simulink model "tutorial25_simscape"  (R2025a)
settings: Solver=VariableStepAuto  StartTime=0.0  StopTime=10  RelTol=1e-3
settings Model: Creator=xing2  LastModifiedBy=xing2

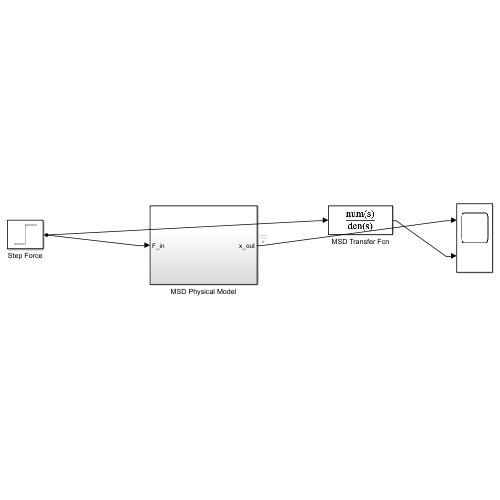
[thumbnail: Simulink's stored preview of the top-level diagram]
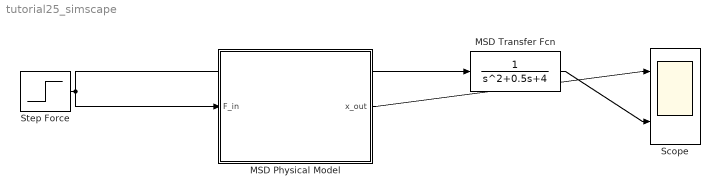
== system tutorial25_simscape ==
  MSD Physical Model : Subsystem
  MSD Transfer Fcn : TransferFcn  Denominator=[1 0.5 4]
  Scope : Scope  NumInputPorts=2
  Step Force : Step  Time=0.5  After=5  SampleTime=0
  wires:
  Step Force/1 -> MSD Physical Model/1(F_in), MSD Transfer Fcn/1
  MSD Physical Model/1(x_out) -> Scope/1
  MSD Transfer Fcn/1 -> Scope/2

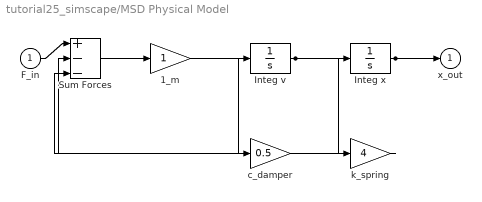
== system tutorial25_simscape/MSD Physical Model ==
  F_in : Inport
  1_m : Gain
  Integ v : Integrator
  Integ x : Integrator
  Sum Forces : Sum  Inputs=|+--
  c_damper : Gain  Gain=0.5
  k_spring : Gain  Gain=4
  x_out : Outport
  wires:
  F_in/1 -> Sum Forces/1
  Sum Forces/1 -> 1_m/1
  1_m/1 -> Integ v/1
  Integ v/1 -> Integ x/1, c_damper/1
  Integ x/1 -> x_out/1, k_spring/1
  c_damper/1 -> Sum Forces/2
  k_spring/1 -> Sum Forces/3
